simulink model "slrtPlantModel"  (R2019a)
settings: configuration reference "plantConfigSet" (kept outside this file)
InitFcn:
  | plantConfigSet = slrt_plant_configset;
model workspace (MATLAB code in the model file):
  | cmdLim = Simulink.Parameter;
  | cmdLim.Value = 15;
  | cmdLim.Description = 'Limit for controlling the maximum surface command angle.';
  | cmdLim.Min = 0;
  | cmdLim.Max = 90;
  | cmdLim.DocUnits = 'deg';
  | 
  | dispGain = Simulink.Parameter;
  | dispGain.Value = 0.75;
  | dispGain.Description = 'Gain applied to the displacement error.';
  | dispGain.Min = 0;
  | dispGain.Max = [];
  | dispGain.DocUnits = 'deg/sec/deg';
  | 
  | dispLim = Simulink.Parameter;
  | dispLim.Value = 30;
  | dispLim.Description = 'Limit for controlling the maximum commanded angle.';
  | dispLim.Min = 0;
  | dispLim.Max = 180;
  | dispLim.DocUnits = 'deg';
  | 
  | intGain = Simulink.Parameter;
  | intGain.Value = 0.5;
  | intGain.Description = 'Gain applied to the integral error.';
  | intGain.Min = 0;
  | intGain.Max = [];
  | intGain.DocUnits = 'deg/sec/deg/sec';
  | 
  | intLim = Simulink.Parameter;
  | intLim.Value = 5;
  | intLim.Description = 'Limit for controlling the maximum commanded angle.';
  | intLim.Min = 0;
  | intLim.Max = 90;
  | intLim.DocUnits = 'deg';
  | 
  | rateGain = Simulink.Parameter;
  | rateGain.Value = 2;
  | rateGain.Description = 'Gain applied to the rate error.';
  | rateGain.Min = 0;
  | rateGain.Max = [];
  | rateGain.DocUnits = 'deg/deg/sec';
  | 
  | rateLim = Simulink.Parameter;
  | rateLim.Value = 6;
  | rateLim.Description = 'Limit for controlling the maximum commanded angle.';
  | rateLim.Min = 0;
  | rateLim.Max = 180;
  | rateLim.DocUnits = 'deg/sec';
  | 
  | hdgGain = Simulink.Parameter;
  | hdgGain.Value = 0.015;
undefined symbols (not defined in the file): env, sensors
libraries: slrtlib x5, xpcrtudplib x3, xpcutilitieslib x2, simulink_extras x2
settings Model: RequirementInfo={} %GIDa_fe9045fd_0412_4b6e_8206_617cc20e6fde  FPTRunName=Active  Creator=mlizarra  LastModifiedBy=gponnu
settings ConfigSetRef: SourceName=plantConfigSet  SourceLocation=Base Workspace

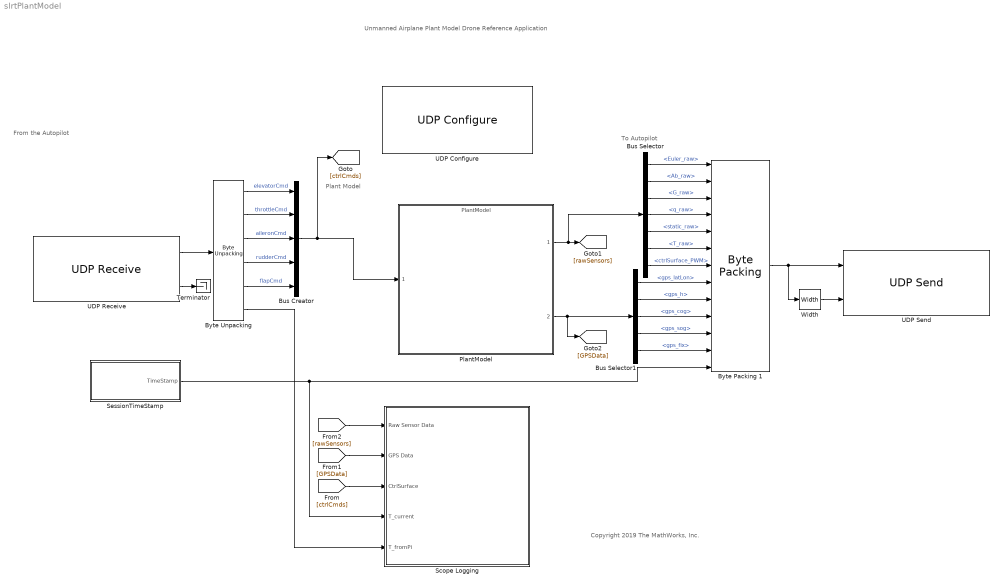
== system slrtPlantModel ==
  note: To Autopilot
  note: From the Autopilot
  note: Unmanned Airplane Plant Model
      |
      | Drone Reference Application
  note: Plant Model
  note: Copyright 2019 The MathWorks, Inc.
  Bus Creator : BusCreator  Inputs=5  OutDataTypeStr=Bus: ctrlCmdsBus
  Bus Selector : BusSelector  OutputSignals=Euler_raw,Ab_raw,G_raw,q_raw,static_raw,T_raw,ctrlSurface_PWM
  Bus Selector1 : BusSelector  OutputSignals=gps_latLon,gps_h,gps_cog,gps_sog,gps_fix
  Byte Packing 1 : xpcutilitieslib/Byte Packing   MaskPackedDataType=uint8  MaskUnpackedDataTypes={['int16'], ['int16'], ['int16'], 'uint16', 'uint16', 'int16', ['int16'], ['single'], 'single', 'single', 'single', 'uint8','double'}  MaskAlignment=1
  "Byte Unpacking " : xpcutilitieslib/Byte Unpacking   MaskUnpackedDataTypes={'single', 'single', 'single', 'single', 'single','double'}  MaskUnpackedDataSizes={1,1,1,1,1,1}  MaskAlignment=1
      settings: SourceProductName=Simulink Real-Time  SourceProductBaseCode=XP
  PlantModel : ModelReference  ModelNameDialog=PlantModel.slx  SimulationMode=Normal  ModelReferenceVersion=1.373
  Scope Logging : Subsystem
  SessionTimeStamp : Subsystem
  Terminator : Terminator
  UDP Configure : xpcrtudplib/UDP Configure  Priority=-1  IpAddress=10.10.10.102  SubnetMask=255.255.255.2  Gateway=0.0.0.0  PciBus=5  PciSlot=0  PciFunction=0  ID=1  tune=0  disable=off  enableMulticast=off  MulticastIpAddress={}  MulticastMask={}
      settings: SourceProductName=Simulink Real-Time  SourceProductBaseCode=XP
  UDP Receive : xpcrtudplib/UDP Receive  ipAddressVal=10.10.10.102  localPort=25000  rcvWidth=28  rcvFmAny=off  fmAddress=10.10.10.6  rcvMulticast=off  multicastAddress=[]  maxUDPQueue=8  sampleTime=-1
      settings: SourceProductName=Simulink Real-Time
  UDP Send : xpcrtudplib/UDP Send  ipAddressVal=Use host-target connection  localPort=25001  toAddress=10.10.10.6  toPort=25001  sampleTime=-1
      settings: SourceProductName=Simulink Real-Time  SourceProductBaseCode=XP
  Width : Width
  wires:
  Bus Creator/1 -> [ctrlCmds], PlantModel/1
  "Byte Unpacking "/1 -> Bus Creator/1  "elevatorCmd"
  "Byte Unpacking "/3 -> Bus Creator/3  "aileronCmd"
  "Byte Unpacking "/2 -> Bus Creator/2  "throttleCmd"
  "Byte Unpacking "/4 -> Bus Creator/4  "rudderCmd"
  "Byte Unpacking "/5 -> Bus Creator/5  "flapCmd"
  Bus Selector/2 -> Byte Packing 1/2  "<Ab_raw>"
  Bus Selector/1 -> Byte Packing 1/1  "<Euler_raw>"
  Bus Selector/3 -> Byte Packing 1/3  "<G_raw>"
  Bus Selector/4 -> Byte Packing 1/4  "<q_raw>"
  Bus Selector/5 -> Byte Packing 1/5  "<static_raw>"
  Bus Selector/6 -> Byte Packing 1/6  "<T_raw>"
  Bus Selector/7 -> Byte Packing 1/7  "<ctrlSurface_PWM>"
  Bus Selector1/1 -> Byte Packing 1/8  "<gps_latLon>"
  Bus Selector1/2 -> Byte Packing 1/9  "<gps_h>"
  Bus Selector1/3 -> Byte Packing 1/10  "<gps_cog>"
  Bus Selector1/4 -> Byte Packing 1/11  "<gps_sog>"
  Bus Selector1/5 -> Byte Packing 1/12  "<gps_fix>"
  Byte Packing 1/1 -> UDP Send/1, Width/1
  Width/1 -> UDP Send/2
  UDP Receive/1 -> "Byte Unpacking "/1
  UDP Receive/2 -> Terminator/1
  [ctrlCmds] -> Scope Logging/3(CtrlSurface)
  [GPSData] -> Scope Logging/2(GPS Data)
  [rawSensors] -> Scope Logging/1(Raw Sensor Data)
  "Byte Unpacking "/6 -> Scope Logging/5(T_fromPi)
  PlantModel/2 -> [GPSData], Bus Selector1/1
  PlantModel/1 -> [rawSensors], Bus Selector/1
  SessionTimeStamp/1(TimeStamp) -> Scope Logging/4(T_current), Byte Packing 1/13

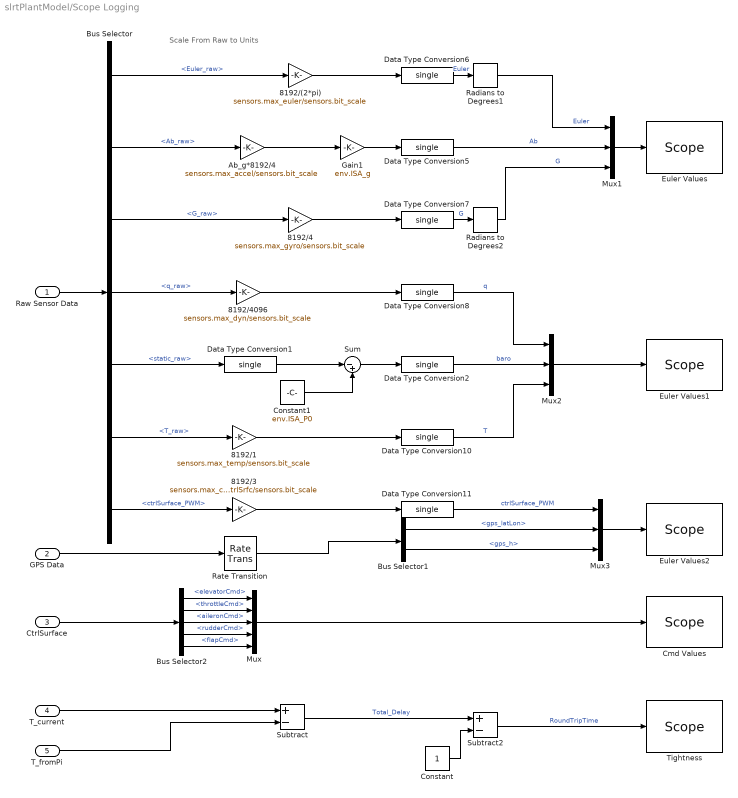
== system slrtPlantModel/Scope Logging ==
  note: Scale From Raw to Units
  Raw Sensor Data : Inport
  GPS Data : Inport  Port=2
  CtrlSurface : Inport  Port=3
  T_current : Inport  Port=4
  T_fromPi : Inport  Port=5
  8192/(2*pi) : Gain  Gain=sensors.max_euler/sensors.bit_scale  OutDataTypeStr=single
      settings: AttributesFormatString=%<Gain>
  8192/1 : Gain  Gain=sensors.max_temp/sensors.bit_scale  OutDataTypeStr=single
      settings: AttributesFormatString=%<Gain>
  8192/3 : Gain  Gain=sensors.max_ctrlSrfc/sensors.bit_scale  OutDataTypeStr=single
      settings: AttributesFormatString=%<Gain>
  8192/4 : Gain  Gain=sensors.max_gyro/sensors.bit_scale  OutDataTypeStr=single
      settings: AttributesFormatString=%<Gain>
  8192/4096 : Gain  Gain=sensors.max_dyn/sensors.bit_scale  OutDataTypeStr=single
      settings: AttributesFormatString=%<Gain>
  Ab_g*8192/4 : Gain  Gain=sensors.max_accel/sensors.bit_scale  OutDataTypeStr=single
      settings: AttributesFormatString=%<Gain>
  Bus Selector : BusSelector  OutputSignals=Euler_raw,Ab_raw,G_raw,q_raw,static_raw,T_raw,ctrlSurface_PWM
  Bus Selector1 : BusSelector  OutputSignals=gps_latLon,gps_h
  Bus Selector2 : BusSelector  OutputSignals=elevatorCmd,throttleCmd,aileronCmd,rudderCmd,flapCmd
  Cmd Values : slrtlib/Displays and Logging/Scope   scopeno=1  scopetype=Target  autostart=on  viewmode=Numerical  formatstr='%15.6f'  grid=on  ylimits=[0,0]  nosamples=250  noprepostsamples=0  interleave=1  triggermode=FreeRun  triggersignal=1  trigsignalfromport=off  triggerlevel=0.0  triggerslope=Either  triggerscope=1  triggersample=0  filename=data.dat  mode=Lazy  writesize=512  autorestart=off  dynamicfilemode=off  maxwritefilesize=512*1024^2
  Constant : Constant
  Constant1 : Constant  Value=env.ISA_P0
      settings: AttributesFormatString=%<Value>
  Data Type Conversion{1..2,5..8,10..11} (8 alike) : DataTypeConversion  OutDataTypeStr=single
  Euler Values : slrtlib/Displays and Logging/Scope   scopeno=2  scopetype=Target  autostart=on  viewmode=Numerical  formatstr='%15.6f'  grid=on  ylimits=[0,0]  nosamples=250  noprepostsamples=0  interleave=1  triggermode=FreeRun  triggersignal=1  trigsignalfromport=off  triggerlevel=0.0  triggerslope=Either  triggerscope=1  triggersample=0  filename=data.dat  mode=Lazy  writesize=512  autorestart=off  dynamicfilemode=off  maxwritefilesize=512*1024^2
  Euler Values1 : slrtlib/Displays and Logging/Scope   scopeno=3  scopetype=Target  autostart=on  viewmode=Numerical  formatstr='%15.6f'  grid=on  ylimits=[0,0]  nosamples=250  noprepostsamples=0  interleave=1  triggermode=FreeRun  triggersignal=1  trigsignalfromport=off  triggerlevel=0.0  triggerslope=Either  triggerscope=1  triggersample=0  filename=data.dat  mode=Lazy  writesize=512  autorestart=off  dynamicfilemode=off  maxwritefilesize=512*1024^2
  Euler Values2 : slrtlib/Displays and Logging/Scope   scopeno=4  scopetype=Target  autostart=on  viewmode=Numerical  formatstr='%15.6f'  grid=on  ylimits=[0,0]  nosamples=250  noprepostsamples=0  interleave=1  triggermode=FreeRun  triggersignal=1  trigsignalfromport=off  triggerlevel=0.0  triggerslope=Either  triggerscope=1  triggersample=0  filename=data.dat  mode=Lazy  writesize=512  autorestart=off  dynamicfilemode=off  maxwritefilesize=512*1024^2
  Gain1 : Gain  Gain=env.ISA_g  OutDataTypeStr=single
      settings: AttributesFormatString=%<Gain>
  Mux : Mux  Inputs=5
  Mux1 : Mux  Inputs=3
  Mux2 : Mux  Inputs=3
  Mux3 : Mux  Inputs=3
  Radians to Degrees1 : simulink_extras/Transformations/Radians to Degrees
  Radians to Degrees2 : simulink_extras/Transformations/Radians to Degrees
  Rate Transition : RateTransition  Deterministic=off
  Subtract : Sum  Inputs=+-
  Subtract2 : Sum  Inputs=+-
  Sum : Sum  Inputs=|-+
  Tightness : slrtlib/Displays and Logging/Scope   scopeno=5  scopetype=Target  autostart=on  viewmode=Numerical  formatstr='%15.6f'  grid=on  ylimits=[0,0]  nosamples=250  noprepostsamples=0  interleave=1  triggermode=FreeRun  triggersignal=1  trigsignalfromport=off  triggerlevel=0.0  triggerslope=Either  triggerscope=1  triggersample=0  filename=data.dat  mode=Lazy  writesize=512  autorestart=off  dynamicfilemode=off  maxwritefilesize=512*1024^2
  wires:
  Mux2/1 -> Euler Values1/1
  Bus Selector/4 -> 8192/4096/1  "<q_raw>"
  Constant1/1 -> Sum/2
  Data Type Conversion8/1 -> Mux2/1  "q"
  Data Type Conversion5/1 -> Mux1/2  "Ab"
  Raw Sensor Data/1 -> Bus Selector/1
  Data Type Conversion10/1 -> Mux2/3  "T"
  Bus Selector/6 -> 8192/1/1  "<T_raw>"
  Data Type Conversion2/1 -> Mux2/2  "baro"
  Data Type Conversion7/1 -> Radians to Degrees2/1  "G"
  Bus Selector/1 -> 8192/(2*pi)/1  "<Euler_raw>"
  Data Type Conversion6/1 -> Radians to Degrees1/1  "Euler"
  Data Type Conversion1/1 -> Sum/1
  Sum/1 -> Data Type Conversion2/1
  Bus Selector/3 -> 8192/4/1  "<G_raw>"
  Gain1/1 -> Data Type Conversion5/1
  Mux1/1 -> Euler Values/1
  8192/4/1 -> Data Type Conversion7/1
  8192/1/1 -> Data Type Conversion10/1
  Ab_g*8192/4/1 -> Gain1/1
  8192/4096/1 -> Data Type Conversion8/1
  Bus Selector/7 -> 8192/3/1  "<ctrlSurface_PWM>"
  8192/(2*pi)/1 -> Data Type Conversion6/1
  Bus Selector/2 -> Ab_g*8192/4/1  "<Ab_raw>"
  Bus Selector/5 -> Data Type Conversion1/1  "<static_raw>"
  8192/3/1 -> Data Type Conversion11/1
  GPS Data/1 -> Rate Transition/1
  Bus Selector1/2 -> Mux3/3  "<gps_h>"
  Mux/1 -> Cmd Values/1
  Bus Selector2/5 -> Mux/5  "<flapCmd>"
  Bus Selector2/4 -> Mux/4  "<rudderCmd>"
  Bus Selector2/2 -> Mux/2  "<throttleCmd>"
  CtrlSurface/1 -> Bus Selector2/1
  Bus Selector2/1 -> Mux/1  "<elevatorCmd>"
  Bus Selector2/3 -> Mux/3  "<aileronCmd>"
  T_current/1 -> Subtract/1
  T_fromPi/1 -> Subtract/2
  Mux3/1 -> Euler Values2/1
  Subtract/1 -> Subtract2/1  "Total_Delay"
  Subtract2/1 -> Tightness/1  "RoundTripTime"
  Constant/1 -> Subtract2/2
  Bus Selector1/1 -> Mux3/2  "<gps_latLon>"
  Data Type Conversion11/1 -> Mux3/1  "ctrlSurface_PWM"
  Radians to Degrees1/1 -> Mux1/1  "Euler"
  Radians to Degrees2/1 -> Mux1/3  "G"
  Rate Transition/1 -> Bus Selector1/1

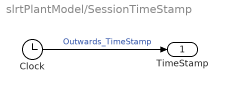
== system slrtPlantModel/SessionTimeStamp ==
  Clock : Clock
  TimeStamp : Outport
  wires:
  Clock/1 -> TimeStamp/1  "Outwards_TimeStamp"
